simulink model "Flex_simulink"  (R2018a)
settings: Solver=FixedStepDiscrete  StartTime=0.0  StopTime=inf  FixedStep=0.00005  RelTol=1e-3  EnableMultiTasking=on
PreLoadFcn:
  | Ts = 0.001;
InitFcn:
  | Ts = 0.001;
values from neighbouring files (symbols this model uses):
  I_limit = 500    [init.m]
libraries: xpcethercatlib x91, simulink x54, slrtlib x2
(part 1 of 2)
settings Model: xpc_rtwmakecfg_data=_xpcethercatlib_  SimulationMode=external  ExtModeTrigDirection=either  ExplicitPartitioning=on  Creator=lab  LastModifiedBy=Mark
settings SolverCC: AutoInsertRateTranBlk=on
settings DataIOCC: Decimation=10  LimitDataPoints=on  SaveFormat=StructureWithTime
settings OptimizationCC: BlockReduction=off  OptimizeBlockIOStorage=off  BufferReuse=off  GlobalBufferReuse=off  ExpressionFolding=off  LocalBlockOutputs=off  OptimizeDataStoreBuffers=off  BusAssignmentInplaceUpdate=off
settings DebuggingCC: UnconnectedInputMsg=none  UnconnectedOutputMsg=none  UnconnectedLineMsg=none
settings HardwareCC: ProdBitPerPointer=32  ProdBitPerSizeT=32  ProdBitPerPtrDiffT=32  ProdLargestAtomicFloat=None  ProdWordSize=32  ProdLongLongMode=on  ProdHWDeviceType=Generic->32-bit x86 compatible
settings RTWCC: SystemTargetFile=slrt.tlc  TemplateMakefile=slrt_default_tmf  Description=Simulink Real-Time  CodeExecutionProfiling=on  RTWCompilerOptimization=on
settings SimulinkRealTimeCC: SupportVariableSizeSignals=on  xPCConcurrentTasks=on

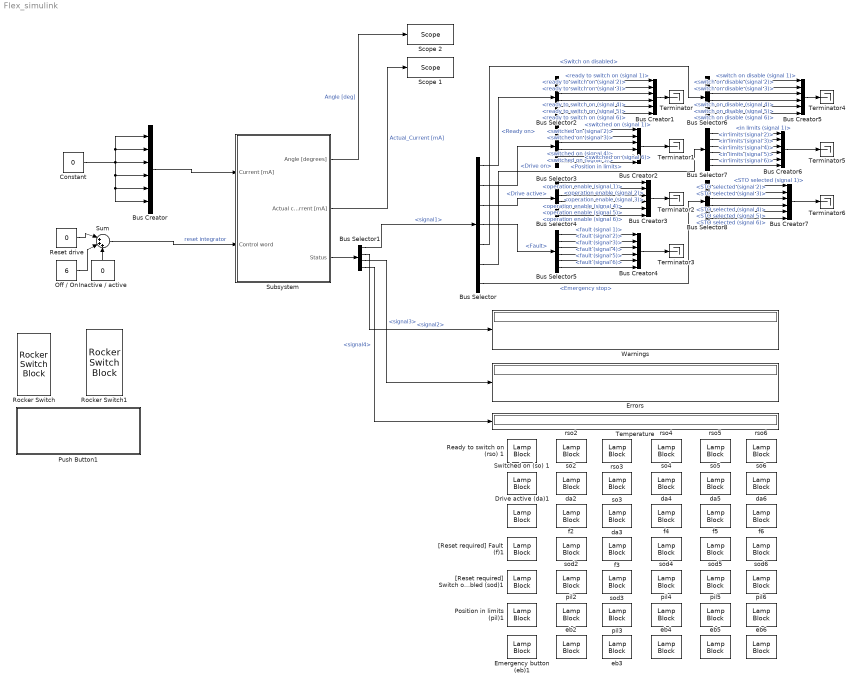
== system Flex_simulink ==
  " da2 " : LampBlock  WebBlockId=1372  LabelPosition=Hide
  " so2 " : LampBlock  WebBlockId=1336  LabelPosition=Hide
  " da4" : LampBlock  WebBlockId=1373  LabelPosition=Hide
  " da5" : LampBlock  WebBlockId=1374  LabelPosition=Hide
  " da6" : LampBlock  WebBlockId=1375  LabelPosition=Hide
  " eb4" : LampBlock  WebBlockId=1402  LabelPosition=Hide
  " eb5" : LampBlock  WebBlockId=1403  LabelPosition=Hide
  " eb6" : LampBlock  WebBlockId=1404  LabelPosition=Hide
  " f4" : LampBlock  WebBlockId=1379  LabelPosition=Hide
  " f5" : LampBlock  WebBlockId=1380  LabelPosition=Hide
  " f6" : LampBlock  WebBlockId=1381  LabelPosition=Hide
  " pil4" : LampBlock  WebBlockId=1397  LabelPosition=Hide
  " pil5" : LampBlock  WebBlockId=1398  LabelPosition=Hide
  " pil6" : LampBlock  WebBlockId=1399  LabelPosition=Hide
  " rso4" : LampBlock  WebBlockId=1325  LabelPosition=Hide
  " so4" : LampBlock  WebBlockId=1333  LabelPosition=Hide
  " so5" : LampBlock  WebBlockId=1334  LabelPosition=Hide
  " so6" : LampBlock  WebBlockId=1335  LabelPosition=Hide
  " sod4" : LampBlock  WebBlockId=1384  LabelPosition=Hide
  " sod5" : LampBlock  WebBlockId=1385  LabelPosition=Hide
  " sod6" : LampBlock  WebBlockId=1386  LabelPosition=Hide
  Bus Creator{,1..7} (8 alike) : BusCreator  Inputs=6
  Bus Selector : BusSelector  OutputSignals=Ready on,Drive on,Drive active,Fault,Switch on disabled,Position in limits,Emergency stop
  Bus Selector1 : BusSelector  OutputSignals=signal1,signal2,signal3,signal4
  Bus Selector2 : BusSelector  OutputSignals=ready to switch on (signal 1),ready to switch on (signal 2),ready to switch on (signal 3),ready to switch on (signal 4),ready to switch on (signal 5),ready to switch on (signal 6)
  Bus Selector3 : BusSelector  OutputSignals=switched on (signal 1),switched on (signal 2),switched on (signal 3),switched on (signal 4),switched on (signal 5),switched on (signal 6)
  Bus Selector4 : BusSelector  OutputSignals=operation enable (signal 1),operation enable (signal 2),operation enable (signal 3),operation enable (signal 4),operation enable (signal 5),operation enable (signal 6)
  Bus Selector5 : BusSelector  OutputSignals=fault (signal 1),fault (signal 2),fault (signal 3),fault (signal 4),fault (signal 5),fault (signal 6)
  Bus Selector6 : BusSelector  OutputSignals=switch on disable (signal 1),switch on disable (signal 2),switch on disable (signal 3),switch on disable (signal 4),switch on disable (signal 5),switch on disable (signal 6)
  Bus Selector7 : BusSelector  OutputSignals=in limits (signal 1),in limits (signal 2),in limits (signal 3),in limits (signal 4),in limits (signal 5),in limits (signal 6)
  Bus Selector8 : BusSelector  OutputSignals=STO selected (signal 1),STO selected (signal 2),STO selected (signal 3),STO selected (signal 4),STO selected (signal 5),STO selected (signal 6)
  Constant : Constant  Value=0
  Drive active (da)1 : LampBlock  WebBlockId=1376
  Emergency button (eb)1 : LampBlock  WebBlockId=1405
  Errors : Display
      settings: Decimation=25
  Inactive / active : Constant  Value=0
  Off / On : Constant  Value=6
  Position in limits (pil)1 : LampBlock  WebBlockId=1400
  Push Button1 : Subsystem  DialogController=hmiCreateDDGDialog  IsWebBlock=on  mask(MWDashboardBlock){webBlockId=c834c18b-4d14-4fd2-a2aa-8470ccae1b8a, webBlockType=pushbutton, ShowInLibBrwoser=on, ShowInitialText=on, HMISrcModelName=Flex_simulink}
      mask prompts: webBlockId "WebBlock Id"; webBlockType "WebBlock Type"; HMISrcModelName "Source Model"
      mask help: SimulinkHMI:dialogs:PushButtonDialogDesc
      mask Help: helpview([docroot '/mapfiles/simulink.map'], 'hmi_push_button')
      mask Display:
      | model = bdroot(gcb);
      | if strcmp(get_param(model,'BlockDiagramType'), 'library')
      |     image([(matlabroot) '/toolbox/simulink/hmi/icons/PushButton.png']);
      | end
  Ready to switch on (rso) 1 : LampBlock  WebBlockId=226
  Reset drive : Constant  Value=0
  Rocker Switch : RockerSwitchBlock  WebBlockId=231
      settings: Values={{'Off', 'On'}, [6 7]}
  Rocker Switch1 : RockerSwitchBlock  WebBlockId=232
      settings: Values={{'Off', 'On'}, [0 8]}
  Scope 1 : slrtlib/Displays and Logging/Scope   scopeno=2  scopetype=Target  autostart=on  viewmode=Numerical  formatstr='%15.6f,%15.6f,%15.6f,%15.6f,%15.6f,%15.6f'  grid=on  ylimits=[500,500]  nosamples=100  noprepostsamples=0  interleave=25  triggermode=FreeRun  triggersignal=1  trigsignalfromport=off  triggerlevel=0.0  triggerslope=Either  triggerscope=1  triggersample=0  filename=data.dat  mode=Lazy  writesize=512  autorestart=off  dynamicfilemode=off  maxwritefilesize=512*1024^2
  Scope 2 : slrtlib/Displays and Logging/Scope   scopeno=1  scopetype=Target  autostart=on  viewmode=Numerical  formatstr='%15.6f,%15.6f,%15.6f,%15.6f,%15.6f,%15.6f'  grid=on  ylimits=[500,500]  nosamples=100  noprepostsamples=0  interleave=25  triggermode=FreeRun  triggersignal=1  trigsignalfromport=off  triggerlevel=0.0  triggerslope=Either  triggerscope=1  triggersample=0  filename=data.dat  mode=Lazy  writesize=512  autorestart=off  dynamicfilemode=off  maxwritefilesize=512*1024^2
  Subsystem : Subsystem
  Sum : Sum  Inputs=|+++
  Switched on (so) 1 : LampBlock  WebBlockId=1338
  Temperature : Display
      settings: Decimation=25
  Terminator{,1..6} (7 alike) : Terminator
  Warnings : Display
      settings: Decimation=25
  "[Reset required] Fault (f)1 " : LampBlock  WebBlockId=1382
  "[Reset required] Switch on disabled (sod)1" : LampBlock  WebBlockId=1387
  da3 : LampBlock  WebBlockId=1377  LabelPosition=Hide
  eb2 : LampBlock  WebBlockId=1406  LabelPosition=Hide
  eb3 : LampBlock  WebBlockId=1407  LabelPosition=Hide
  f2 : LampBlock  WebBlockId=1378  LabelPosition=Hide
  f3 : LampBlock  WebBlockId=1383  LabelPosition=Hide
  pil2 : LampBlock  WebBlockId=1396  LabelPosition=Hide
  pil3 : LampBlock  WebBlockId=1401  LabelPosition=Hide
  rso2 : LampBlock  WebBlockId=1323  LabelPosition=Hide
  rso3 : LampBlock  WebBlockId=1324  LabelPosition=Hide
  rso5 : LampBlock  WebBlockId=1326  LabelPosition=Hide
  rso6 : LampBlock  WebBlockId=1327  LabelPosition=Hide
  so3 : LampBlock  WebBlockId=1337  LabelPosition=Hide
  sod2 : LampBlock  WebBlockId=1388  LabelPosition=Hide
  sod3 : LampBlock  WebBlockId=1389  LabelPosition=Hide
  wires:
  Subsystem/2(Actual current [mA]) -> Scope 1/1  "Actual_Current [mA]"
  Bus Selector/1 -> Bus Selector2/1  "<Ready on>"
  Bus Selector/2 -> Bus Selector3/1  "<Drive on>"
  Bus Selector/3 -> Bus Selector4/1  "<Drive active>"
  Bus Selector/4 -> Bus Selector5/1  "<Fault>"
  Bus Selector/5 -> Bus Selector6/1  "<Switch on disabled>"
  Bus Selector/6 -> Bus Selector7/1  "<Position in limits>"
  Bus Selector/7 -> Bus Selector8/1  "<Emergency stop>"
  Reset drive/1 -> Sum/1
  Off / On/1 -> Sum/2
  Inactive / active/1 -> Sum/3
  Sum/1 -> Subsystem/2(Control word)  "reset integrator"
  Subsystem/1(Angle [degrees]) -> Scope 2/1  "Angle [deg]"
  Constant/1 -> Bus Creator/6, Bus Creator/5, Bus Creator/4, Bus Creator/3, Bus Creator/2, Bus Creator/1
  Bus Creator/1 -> Subsystem/1(Current [mA])
  Subsystem/3(Status) -> Bus Selector1/1
  Bus Selector1/4 -> Temperature/1  "<signal4>"
  Bus Selector1/3 -> Errors/1  "<signal3>"
  Bus Selector1/2 -> Warnings/1  "<signal2>"
  Bus Selector1/1 -> Bus Selector/1  "<signal1>"
  Bus Selector2/1 -> Bus Creator1/1  "<ready to switch on (signal 1)>"
  Bus Selector2/2 -> Bus Creator1/2  "<ready to switch on (signal 2)>"
  Bus Selector2/3 -> Bus Creator1/3  "<ready to switch on (signal 3)>"
  Bus Selector2/4 -> Bus Creator1/4  "<ready to switch on (signal 4)>"
  Bus Selector2/5 -> Bus Creator1/5  "<ready to switch on (signal 5)>"
  Bus Selector2/6 -> Bus Creator1/6  "<ready to switch on (signal 6)>"
  Bus Creator1/1 -> Terminator/1
  Bus Selector3/2 -> Bus Creator2/2  "<switched on (signal 2)>"
  Bus Selector3/1 -> Bus Creator2/1  "<switched on (signal 1)>"
  Bus Selector3/5 -> Bus Creator2/5  "<switched on (signal 5)>"
  Bus Creator2/1 -> Terminator1/1
  Bus Selector3/4 -> Bus Creator2/4  "<switched on (signal 4)>"
  Bus Selector3/6 -> Bus Creator2/6  "<switched on (signal 6)>"
  Bus Selector3/3 -> Bus Creator2/3  "<switched on (signal 3)>"
  Bus Selector4/4 -> Bus Creator3/4  "<operation enable (signal 4)>"
  Bus Selector4/6 -> Bus Creator3/6  "<operation enable (signal 6)>"
  Bus Creator3/1 -> Terminator2/1
  Bus Selector4/5 -> Bus Creator3/5  "<operation enable (signal 5)>"
  Bus Selector4/1 -> Bus Creator3/1  "<operation enable (signal 1)>"
  Bus Selector4/2 -> Bus Creator3/2  "<operation enable (signal 2)>"
  Bus Selector4/3 -> Bus Creator3/3  "<operation enable (signal 3)>"
  Bus Selector5/4 -> Bus Creator4/4  "<fault (signal 4)>"
  Bus Selector5/6 -> Bus Creator4/6  "<fault (signal 6)>"
  Bus Creator4/1 -> Terminator3/1
  Bus Selector5/5 -> Bus Creator4/5  "<fault (signal 5)>"
  Bus Selector5/1 -> Bus Creator4/1  "<fault (signal 1)>"
  Bus Selector5/2 -> Bus Creator4/2  "<fault (signal 2)>"
  Bus Selector5/3 -> Bus Creator4/3  "<fault (signal 3)>"
  Bus Selector6/4 -> Bus Creator5/4  "<switch on disable (signal 4)>"
  Bus Selector6/6 -> Bus Creator5/6  "<switch on disable (signal 6)>"
  Bus Creator5/1 -> Terminator4/1
  Bus Selector6/5 -> Bus Creator5/5  "<switch on disable (signal 5)>"
  Bus Selector6/1 -> Bus Creator5/1  "<switch on disable (signal 1)>"
  Bus Selector6/2 -> Bus Creator5/2  "<switch on disable (signal 2)>"
  Bus Selector6/3 -> Bus Creator5/3  "<switch on disable (signal 3)>"
  Bus Selector7/4 -> Bus Creator6/4  "<in limits (signal 4)>"
  Bus Selector7/6 -> Bus Creator6/6  "<in limits (signal 6)>"
  Bus Creator6/1 -> Terminator5/1
  Bus Selector7/5 -> Bus Creator6/5  "<in limits (signal 5)>"
  Bus Selector7/1 -> Bus Creator6/1  "<in limits (signal 1)>"
  Bus Selector7/2 -> Bus Creator6/2  "<in limits (signal 2)>"
  Bus Selector7/3 -> Bus Creator6/3  "<in limits (signal 3)>"
  Bus Selector8/4 -> Bus Creator7/4  "<STO selected (signal 4)>"
  Bus Selector8/6 -> Bus Creator7/6  "<STO selected (signal 6)>"
  Bus Creator7/1 -> Terminator6/1
  Bus Selector8/5 -> Bus Creator7/5  "<STO selected (signal 5)>"
  Bus Selector8/1 -> Bus Creator7/1  "<STO selected (signal 1)>"
  Bus Selector8/2 -> Bus Creator7/2  "<STO selected (signal 2)>"
  Bus Selector8/3 -> Bus Creator7/3  "<STO selected (signal 3)>"

== system Flex_simulink/Push Button1 ==
